simulink model "AirTableModel"  (R2021a)
settings: Solver=FixedStepAuto  StartTime=0.0  StopTime=endTime  FixedStep=dynamicsRate  RelTol=1e-3  EnableMultiTasking=on
InitFcn:
  | loadThrusterData
  | loadSensorData
values from neighbouring files (symbols this model uses):
  AccelIIR_Den = [1.000000000000000  -1.561018075800718   0.641351538057563]    [loadSensorData.m]
  AccelIIR_Num = [0.020083365564211   0.040166731128423   0.020083365564211]    [loadSensorData.m]
  cameraVec = [1 0 0]    [loadSensorData.m]
  controlRate = 0.025    [loadBusData.m]
  controlType = 1    [loadBusData.m]    (also in loadControlData.m = 2)
  dynamicsRate = 0.005    [loadBusData.m]
  finalRangeAttitude = [0 0 90]*dtr    [loadGuidanceData.m]
  finalRangeValue = 0.25    [loadGuidanceData.m]
  initialCovariance = diag([999999 999999 999999 999999 999999 999999])    [loadSensorData.m]
  initialNavState = [initialState + [0.01 -0.01 1e-3 0 0 1e-3]]    [loadSensorData.m]
  Kd = [x(4) x(5) 0 0 0 x(6)]    [executeSim.m]    (also in loadBusData.m = [500.0000  501.0938 0 0 0 18.4778]; loadControlData.m = [80 80 0 0 0 5] .*[.2 .2  0 0 0 .1]; planarPIDControl.m = [kd(1) 0 0; 0 kd(2) 0; 0 0 kd(3)])
  Ki = [x(7) x(8) 0 0 0 x(9)]    [executeSim.m]    (also in loadBusData.m = [1.0000    1.0313   0 0 0 58.1181]; loadControlData.m = [4  4  0 0 0 1] .*[1   1  0 0 0 .5]; planarPIDControl.m = [ki(1) 0 0; 0 ki(2) 0; 0 0 ki(3)])
  Kp = [x(1) x(2) 0 0 0 x(3)]    [executeSim.m]    (also in loadBusData.m = [500.0000  246.1321 0 0 0 50.1701]; loadControlData.m = [70 70 0 0 0 20].*[.2 .2  0 0 0 .25]; planarPIDControl.m = [kp(1) 0 0; 0 kp(2) 0; 0 0 kp(3)])
  M_Tracker_To_Body = [1 0 0; 0 1 0; 0 0 1]    [loadSensorData.m]
  measurementNoise = [1 .0873 0.0017 2].* [.01 1 1 .01]    [loadSensorData.m]
  processNoise = 0    [loadSensorData.m]
  R_Tracker_To_ECEF = [0 0 0]    [loadSensorData.m]
  rangeSensorAngBody = [0; 90*dtr; 180*dtr; 270*dtr]    [loadSensorData.m]
  rangeSensorFOV = [0*dtr; 0*dtr; 0*dtr; 0*dtr]    [loadSensorData.m]
  rangeSensorIdx = 1    [loadGuidanceData.m]
  SMGains = x    [executeSim.m]    (also in loadBusData.m = [2.0801    3.0489    8.9333    4.9881    3.0029    9.5293   ; loadControlData.m = [3.5078    3.9888    6.3119    1.8214    4.7749    7.3059   )
  useRangeGuid = 0    [loadGuidanceData.m]
  VelIIR_Den = [1.000000000000000  -1.944477657767094   0.945977936232282]    [loadSensorData.m]
  VelIIR_Num = [0.375069616296964   0.750139232593927   0.375069616296964]*1e-3    [loadSensorData.m]
  wallBounds = [wallA; wallB; wallC; wallD]    [loadSensorData.m]
undefined symbols (not defined in the file or in its folder): initialState, navType, PPGains, rangeSensorLocBody, refIdx, targetVec
libraries: simulink x25
(part 1 of 2)
settings Model: SimulationMode=external  Creator=Andy  LastModifiedBy=Andy
settings SolverCC: AlgebraicLoopSolver=TrustRegion  PositivePriorityOrder=on
settings DataIOCC: Decimation=5  SaveFormat=StructureWithTime  ReturnWorkspaceOutputs=off
settings OptimizationCC: EnhancedBackFolding=on  PassReuseOutputArgsAs=Individual arguments  ZeroExternalMemoryAtStartup=off  ZeroInternalMemoryAtStartup=off  MaxStackSize=1024  OptimizeBlockOrder=speed  DifferentSizesBufferReuse=on  OptimizationCustomize=off  EfficientTunableParamExpr=on
settings DebuggingCC: ParameterTunabilityLossMsg=error  SFMachineParentedDataDiag=warning  ArithmeticOperatorsInVariantConditions=warning
settings HardwareCC: ProdBitPerPointer=32  ProdBitPerSizeT=32  ProdBitPerPtrDiffT=32  ProdLargestAtomicInteger=Long  ProdLargestAtomicFloat=Double  ProdWordSize=32  ProdHWDeviceType=ARM Compatible->ARM Cortex
settings ModelReferenceCC: ModelReferenceNumInstancesAllowed=Single
settings SFSimCC: CustomCodeUndefinedFunction=UseInterfaceOnly  SimTargetLang=C++
settings RTWCC: SystemTargetFile=ert.tlc  HardwareBoard=Raspberry Pi  TLCOptions="-aInlineSetEventsForThisBaseRateFcn=TLC_TRUE -aSuppressMultiTaskScheduler=TLC_FALSE  -aRateBasedStepFcn=0"  GenCodeOnly=on  TemplateMakefile=ert_default_tmf  GenerateReport=on  Toolchain=GNU GCC Embedded Linux  BuildConfiguration=Faster Runs  IncludeHyperlinkInReport=on  LaunchReport=on  TargetLang=C++  GenerateTraceInfo=on  GenerateTraceReport=on  GenerateTraceReportSl=on  GenerateTraceReportSf=on  GenerateTraceReportEml=on
settings CodeAppCC: ForceParamTrailComments=on  IgnoreCustomStorageClasses=off  OperatorAnnotations=on  SimulinkDataObjDesc=on  SFDataObjDesc=on  InsertBlockDesc=on
settings ERTTargetCC: TargetLangStandard=C++03 (ISO)  UtilityFuncGeneration=Shared location  MatFileLogging=on  CodeInterfacePackaging=C++ class  SupportVariableSizeSignals=on  MultiInstanceErrorCode=Warning  RootIOFormat=Structure reference

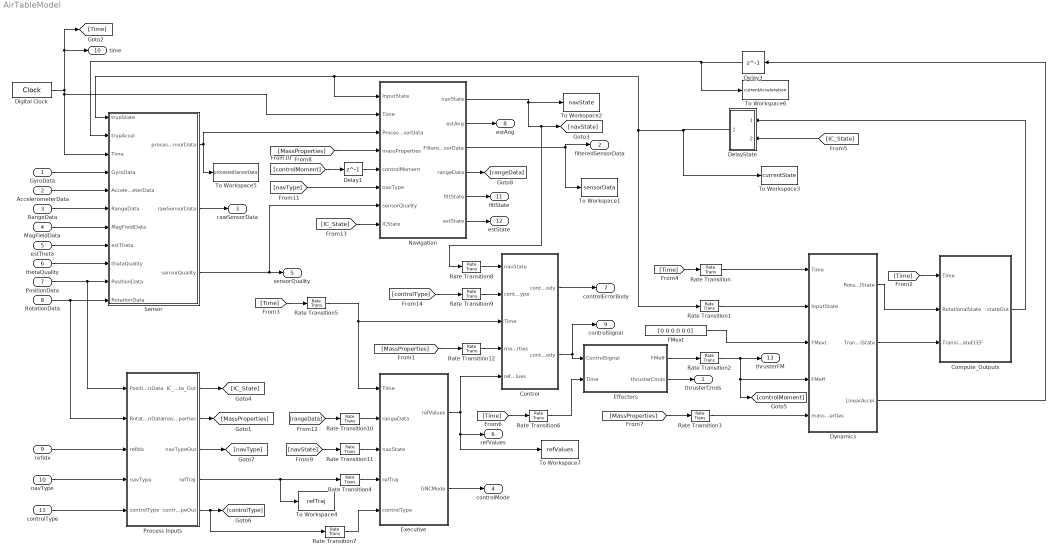
== system AirTableModel ==
  GyroData : Inport  Interpolate=off
  AccelerometerData : Inport  Port=2  Interpolate=off
  RangeData : Inport  Port=3  OutDataTypeStr=int32  Interpolate=off
  MagFieldData : Inport  Port=4  Interpolate=off
  estTheta : Inport  Port=5  OutDataTypeStr=double  PortDimensions=1  Interpolate=off
  thetaQuality : Inport  Port=6  OutDataTypeStr=double  PortDimensions=[1]  Interpolate=off
  PositionData : Inport  Port=7  OutDataTypeStr=double  PortDimensions=3  Interpolate=off
  RotationData : Inport  Port=8  OutDataTypeStr=double  PortDimensions=3  Interpolate=off
  refIdx : Inport  Port=9  OutDataTypeStr=uint8  PortDimensions=1  Interpolate=off
  navType : Inport  Port=10  OutDataTypeStr=uint8  PortDimensions=1  Interpolate=off
  controlType : Inport  Port=11  OutDataTypeStr=uint8  PortDimensions=1  Interpolate=off
  Compute_Outputs : Subsystem
  Control : Subsystem
  Delay1 : Delay  DelayLength=1
  Delay3 : Delay  DelayLength=1
  DelayState : Subsystem
  Digital Clock : DigitalClock  SampleTime=dynamicsRate
  Dynamics : Subsystem  TreatAsAtomicUnit=on  SystemSampleTime=dynamicsRate
      settings: MinAlgLoopOccurrences=on
  Effectors : Subsystem  TreatAsAtomicUnit=on
  Executive : Subsystem  TreatAsAtomicUnit=on  SystemSampleTime=controlRate
  FMext : Constant  Value=[0 0 0 0 0 0]
  Navigation : Subsystem
  Process Inputs : Subsystem
  Rate Transition{,1..3} (4 alike) : RateTransition  OutPortSampleTime=dynamicsRate
  Rate Transition{4..12} (9 alike) : RateTransition  OutPortSampleTime=controlRate
  Sensor : Subsystem
  To Workspace1 : ToWorkspace  VariableName=sensorData  SaveFormat=Timeseries  SampleTime=-1
  To Workspace2 : ToWorkspace  VariableName=navState  SaveFormat=Timeseries  SampleTime=-1
  To Workspace3 : ToWorkspace  VariableName=currentState  SaveFormat=Timeseries  SampleTime=-1
  To Workspace4 : ToWorkspace  VariableName=refTraj  SaveFormat=Timeseries  SampleTime=-1
  To Workspace5 : ToWorkspace  VariableName=processedSensorData  SaveFormat=Timeseries  SampleTime=-1
  To Workspace6 : ToWorkspace  VariableName=currentAcceleration  SaveFormat=Timeseries  SampleTime=-1
  To Workspace7 : ToWorkspace  VariableName=refValues  SaveFormat=Timeseries  SampleTime=-1
  thrusterCmds : Outport  VectorParamsAs1DForOutWhenUnconnected=off
  filteredSensorData : Outport  Port=2  OutDataTypeStr=double  VectorParamsAs1DForOutWhenUnconnected=off
  rawSensorData : Outport  Port=3  OutDataTypeStr=double  VectorParamsAs1DForOutWhenUnconnected=off
  controlMode : Outport  Port=4  VectorParamsAs1DForOutWhenUnconnected=off
  sensorQuality : Outport  Port=5  VectorParamsAs1DForOutWhenUnconnected=off
  refValues : Outport  Port=6  OutDataTypeStr=double  VectorParamsAs1DForOutWhenUnconnected=off
  controlErrorBody : Outport  Port=7  VectorParamsAs1DForOutWhenUnconnected=off
  estAng : Outport  Port=8  VectorParamsAs1DForOutWhenUnconnected=off
  controlSignal : Outport  Port=9  VectorParamsAs1DForOutWhenUnconnected=off
  time : Outport  Port=10  VectorParamsAs1DForOutWhenUnconnected=off
  filtState : Outport  Port=11  OutDataTypeStr=double  VectorParamsAs1DForOutWhenUnconnected=off
  estState : Outport  Port=12  OutDataTypeStr=double  VectorParamsAs1DForOutWhenUnconnected=off
  thrusterFM : Outport  Port=13  VectorParamsAs1DForOutWhenUnconnected=off
  wires:
  Digital Clock/1 -> Navigation/2(Time), Sensor/3(Time), [Time], time/1
  FMext/1 -> Dynamics/3(FMext)
  Control/2(controlSignalBody) -> controlSignal/1, Effectors/1(ControlSignal)
  Dynamics/1(RotationalState) -> Compute_Outputs/2(RotationalState)
  Rate Transition/1 -> Dynamics/1(Time)
  Rate Transition1/1 -> Dynamics/2(InputState)
  Effectors/1(FMeff) -> Rate Transition2/1
  Rate Transition2/1 -> [controlMoment], Dynamics/4(FMeff), thrusterFM/1
  Rate Transition3/1 -> Dynamics/5(massProperties)
  Rate Transition5/1 -> Executive/1(Time), Control/3(Time)
  Rate Transition6/1 -> Effectors/2(Time)
  Dynamics/2(TranslationalState) -> Compute_Outputs/3(TranslationalStateECEF)
  Compute_Outputs/1(stateOut) -> DelayState/1(In4)
  [IC_State] -> DelayState/2(In12)
  DelayState/1(Out4) -> To Workspace3/1, Rate Transition1/1, Navigation/1(InputState), Sensor/1(trueState)
  [Time] -> Compute_Outputs/1(Time)
  Rate Transition8/1 -> Control/1(navState)
  Effectors/2(thrusterCmds) -> thrusterCmds/1
  GyroData/1 -> Sensor/4(GyroData)
  AccelerometerData/1 -> Sensor/5(AccelerometerData)
  RangeData/1 -> Sensor/6(RangeData)
  Executive/1(refValues) -> Control/5(refValues), To Workspace7/1, refValues/1
  Rate Transition11/1 -> Executive/3(navState)
  [Time] -> Rate Transition5/1
  MagFieldData/1 -> Sensor/7(MagFieldData)
  Navigation/1(navState) -> Rate Transition8/1, [navState], To Workspace2/1
  [Time] -> Rate Transition/1
  [Time] -> Rate Transition6/1
  Rate Transition12/1 -> Control/4(massProperties)
  [MassProperties] -> Rate Transition12/1
  [MassProperties] -> Rate Transition3/1
  estTheta/1 -> Sensor/8(estTheta)
  thetaQuality/1 -> Sensor/9(thetaQuality)
  PositionData/1 -> Sensor/10(PositionData), Process Inputs/1(PositionData)
  RotationData/1 -> Process Inputs/2(RotationData), Sensor/11(RotationData)
  Sensor/1(processedSensorData) -> Navigation/3(ProcessedSensorData), To Workspace5/1
  Sensor/2(rawSensorData) -> rawSensorData/1
  [navState] -> Rate Transition11/1
  Rate Transition4/1 -> Executive/4(refTraj)
  Sensor/3(sensorQuality) -> sensorQuality/1, Navigation/7(sensorQuality)
  Control/1(controlErrorBody) -> controlErrorBody/1
  Navigation/2(estAng) -> estAng/1
  Dynamics/3(LinearAccel) -> Delay3/1
  Delay3/1 -> To Workspace6/1, Sensor/2(trueAccel)
  Navigation/3(FilteredSensorData) -> To Workspace1/1, filteredSensorData/1
  [MassProperties] -> Navigation/4(massProperties)
  [controlMoment] -> Delay1/1
  Delay1/1 -> Navigation/5(controlMoment)
  Navigation/5(flttState) -> filtState/1
  Navigation/6(estState) -> estState/1
  [navType] -> Navigation/6(navType)
  Process Inputs/4(refTraj) -> To Workspace4/1, Rate Transition4/1
  refIdx/1 -> Process Inputs/3(refIdx)
  navType/1 -> Process Inputs/4(navType)
  Process Inputs/2(massProperties) -> [MassProperties]
  Process Inputs/3(navTypeOut) -> [navType]
  Process Inputs/1(IC_State_Out) -> [IC_State]
  Rate Transition10/1 -> Executive/2(rangeData)
  Navigation/4(rangeData) -> [rangeData]
  [rangeData] -> Rate Transition10/1
  Executive/2(GNCMode) -> controlMode/1
  [IC_State] -> Navigation/8(ICState)
  [controlType] -> Rate Transition9/1
  controlType/1 -> Process Inputs/5(controlType)
  Process Inputs/5(controlTypeOut) -> Rate Transition7/1, [controlType]
  Rate Transition7/1 -> Executive/5(controlType)
  Rate Transition9/1 -> Control/2(controlType)

== system AirTableModel/Compute_Outputs ==
  Time : Inport
  RotationalState : Inport  Port=2
  TranslationalStateECEF : Inport  Port=3
  Bus Creator2 : BusCreator  Inputs=2  OutDataTypeStr=Bus: TranStateBodyBus
      settings: InheritFromInputs=off
  Bus Creator3 : BusCreator  Inputs=3  OutDataTypeStr=Bus: FullStateBus
      settings: InheritFromInputs=off
  Bus Selector : BusSelector  OutputSignals=ECEF_To_Body_Quat
  Bus Selector1 : BusSelector  OutputSignals=R_Sys_ECEF,V_Sys_ECEF
  Rotate_Vector : MATLAB Function  TreatAsAtomicUnit=on
  Rotate_Vector1 : MATLAB Function  TreatAsAtomicUnit=on
  Terminator1 : Terminator
  Terminator2 : Terminator
  To Workspace1 : ToWorkspace  VariableName=stateOutBus  SaveFormat=Timeseries  SampleTime=-1
  computeRangeData : Subsystem  Commented=on
  stateOut : Outport  VectorParamsAs1DForOutWhenUnconnected=off
  wires:
  RotationalState/1 -> Bus Creator3/1, Bus Selector/1
  Rotate_Vector/1(vOut) -> Bus Creator2/1
  Rotate_Vector1/1(vOut) -> Bus Creator2/2
  TranslationalStateECEF/1 -> Bus Creator3/2, Bus Selector1/1
  Bus Selector1/1 -> Rotate_Vector/1(vIn)  "<R_Sys_ECEF>"
  Bus Creator3/1 -> stateOut/1, To Workspace1/1, computeRangeData/2(In1)
  Time/1 -> computeRangeData/1(Time)
  Bus Selector/1 -> Rotate_Vector1/2(quat), [ECEF_To_Body_Quat]  "<ECEF_To_Body_Quat>"
  [ECEF_To_Body_Quat] -> Rotate_Vector/2(quat)
  Bus Selector1/2 -> Rotate_Vector1/1(vIn)  "<V_Sys_ECEF>"
  computeRangeData/1(range) -> Terminator1/1
  computeRangeData/2(rangeArray) -> Terminator2/1
  Bus Creator2/1 -> Bus Creator3/3

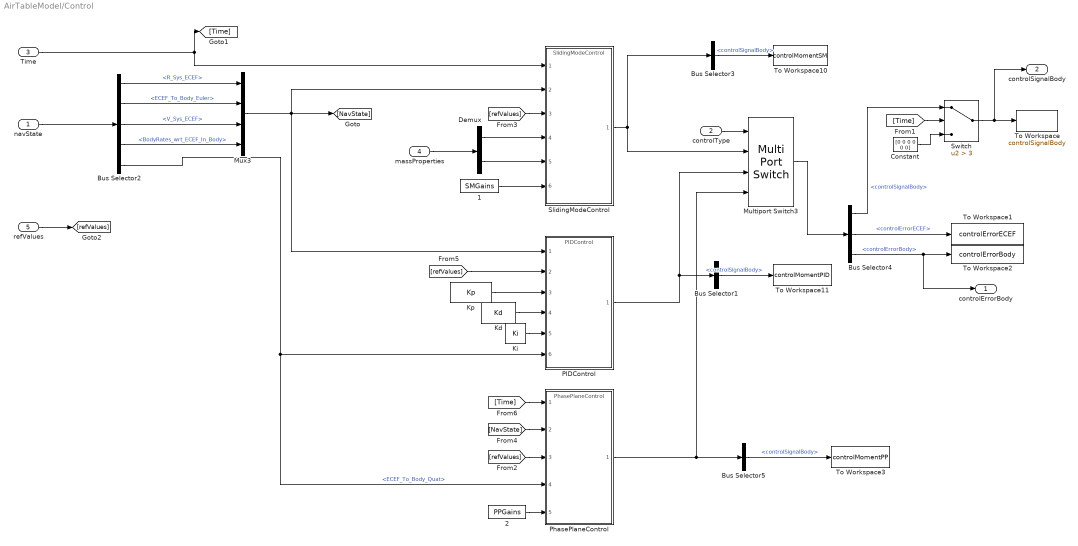
== system AirTableModel/Control ==
  navState : Inport
  controlType : Inport  Port=2
  Time : Inport  Port=3
  massProperties : Inport  Port=4
  refValues : Inport  Port=5
  " 1" : Constant  Value=SMGains
  " 2" : Constant  Value=PPGains
  Bus Selector1 : BusSelector  OutputSignals=controlSignalBody
  Bus Selector2 : BusSelector  OutputSignals=TranState_ECEF.R_Sys_ECEF,RotState_Body_ECEF.ECEF_To_Body_Euler,TranState_ECEF.V_Sys_ECEF,RotState_Body_ECEF.BodyRates_wrt_ECEF_In_Body,RotState_Body_ECEF.ECEF_To_Body_Quat
  Bus Selector3 : BusSelector  OutputSignals=controlSignalBody
  Bus Selector4 : BusSelector  OutputSignals=controlSignalBody,controlErrorECEF,controlErrorBody
  Bus Selector5 : BusSelector  OutputSignals=controlSignalBody
  Constant : Constant  Value=[0 0 0 0 0 0]
  Demux : Demux  Outputs=2
  Kd : Constant  Value=Kd
  Ki : Constant  Value=Ki
  Kp : Constant  Value=Kp
  Multiport Switch3 : MultiPortSwitch
  Mux3 : Mux
  PIDControl : ModelReference  ModelNameDialog=PIDControl  SimulationMode=Normal  ModelReferenceVersion=6.1
  PhasePlaneControl : ModelReference  ModelNameDialog=PhasePlaneControl  SimulationMode=Normal  ModelReferenceVersion=6.20
  SlidingModeControl : ModelReference  ModelNameDialog=SlidingModeControl  SimulationMode=Normal  ModelReferenceVersion=6.1
  Switch : Switch  Criteria=u2 > Threshold  Threshold=3
  To Workspace : ToWorkspace  VariableName=controlSignalBody  SaveFormat=Timeseries  SampleTime=-1
  To Workspace1 : ToWorkspace  VariableName=controlErrorECEF  SaveFormat=Timeseries  SampleTime=-1
  To Workspace10 : ToWorkspace  VariableName=controlMomentSM  SaveFormat=Timeseries  SampleTime=-1
  To Workspace11 : ToWorkspace  VariableName=controlMomentPID  SaveFormat=Timeseries  SampleTime=-1
  To Workspace2 : ToWorkspace  VariableName=controlErrorBody  SaveFormat=Timeseries  SampleTime=-1
  To Workspace3 : ToWorkspace  VariableName=controlMomentPP  SaveFormat=Timeseries  SampleTime=-1
  controlErrorBody : Outport  VectorParamsAs1DForOutWhenUnconnected=off
  controlSignalBody : Outport  Port=2  VectorParamsAs1DForOutWhenUnconnected=off
  wires:
  Mux3/1 -> PIDControl/1, [NavState], SlidingModeControl/2
  navState/1 -> Bus Selector2/1
  Bus Selector2/1 -> Mux3/1  "<R_Sys_ECEF>"
  Bus Selector2/2 -> Mux3/2  "<ECEF_To_Body_Euler>"
  Bus Selector2/3 -> Mux3/3  "<V_Sys_ECEF>"
  Bus Selector2/4 -> Mux3/4  "<BodyRates_wrt_ECEF_In_Body>"
  Kp/1 -> PIDControl/3
  Kd/1 -> PIDControl/4
  Ki/1 -> PIDControl/5
  Demux/2 -> SlidingModeControl/5
  SlidingModeControl/1 -> Bus Selector3/1, Multiport Switch3/2
  controlType/1 -> Multiport Switch3/1
  PIDControl/1 -> Bus Selector1/1, Multiport Switch3/3
  Multiport Switch3/1 -> Bus Selector4/1
  Bus Selector4/1 -> Switch/1  "<controlSignalBody>"
  Bus Selector4/2 -> To Workspace1/1  "<controlErrorECEF>"
  Bus Selector4/3 -> controlErrorBody/1, To Workspace2/1  "<controlErrorBody>"
  Bus Selector1/1 -> To Workspace11/1  "<controlSignalBody>"
  Bus Selector3/1 -> To Workspace10/1  "<controlSignalBody>"
  " 1"/1 -> SlidingModeControl/6
  Demux/1 -> SlidingModeControl/4
  massProperties/1 -> Demux/1
  Time/1 -> [Time], SlidingModeControl/1
  [refValues] -> SlidingModeControl/3
  [refValues] -> PIDControl/2
  Bus Selector2/5 -> PIDControl/6, PhasePlaneControl/4  "<ECEF_To_Body_Quat>"
  [Time] -> Switch/2
  Switch/1 -> controlSignalBody/1, To Workspace/1
  Constant/1 -> Switch/3
  refValues/1 -> [refValues]
  [refValues] -> PhasePlaneControl/3
  [NavState] -> PhasePlaneControl/2
  " 2"/1 -> PhasePlaneControl/5
  [Time] -> PhasePlaneControl/1
  Bus Selector5/1 -> To Workspace3/1  "<controlSignalBody>"
  PhasePlaneControl/1 -> Multiport Switch3/4, Bus Selector5/1

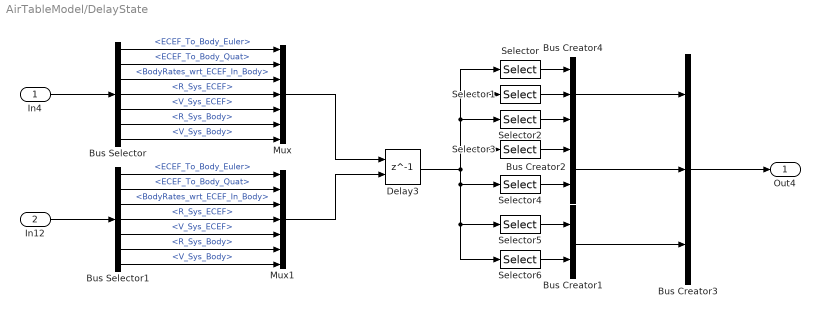
== system AirTableModel/DelayState ==
  In4 : Inport
  In12 : Inport  Port=2
  Bus Creator1 : BusCreator  Inputs=2  OutDataTypeStr=Bus: TranStateBodyBus
      settings: InheritFromInputs=off
  Bus Creator2 : BusCreator  Inputs=2  OutDataTypeStr=Bus: TranStateECEFBus
      settings: InheritFromInputs=off
  Bus Creator3 : BusCreator  Inputs=3  OutDataTypeStr=Bus: FullStateBus
      settings: InheritFromInputs=off
  Bus Creator4 : BusCreator  Inputs=3  OutDataTypeStr=Bus: RotStateBodyECEFBus
      settings: InheritFromInputs=off
  Bus Selector : BusSelector  OutputSignals=RotState_Body_ECEF.ECEF_To_Body_Euler,RotState_Body_ECEF.ECEF_To_Body_Quat,RotState_Body_ECEF.BodyRates_wrt_ECEF_In_Body,TranState_ECEF.R_Sys_ECEF,TranState_ECEF.V_Sys_ECEF,TranState_Body.R_Sys_Body,TranState_Body.V_Sys_Body
  Bus Selector1 : BusSelector  OutputSignals=RotState_Body_ECEF.ECEF_To_Body_Euler,RotState_Body_ECEF.ECEF_To_Body_Quat,RotState_Body_ECEF.BodyRates_wrt_ECEF_In_Body,TranState_ECEF.R_Sys_ECEF,TranState_ECEF.V_Sys_ECEF,TranState_Body.R_Sys_Body,TranState_Body.V_Sys_Body
  Delay3 : Delay  DelayLength=1  InitialConditionSource=Input port
      settings: InputPortMap=u0,p4
  Mux : Mux  Inputs=7
  Mux1 : Mux  Inputs=7
  Selector : Selector  InputPortWidth=22  IndexOptions=Index vector (dialog)  Indices=[1:3]  OutputSizes=1
  Selector1 : Selector  InputPortWidth=22  IndexOptions=Index vector (dialog)  Indices=[4:7]  OutputSizes=1
  Selector2 : Selector  InputPortWidth=22  IndexOptions=Index vector (dialog)  Indices=[8:10]  OutputSizes=1
  Selector3 : Selector  InputPortWidth=22  IndexOptions=Index vector (dialog)  Indices=[11:13]  OutputSizes=1
  Selector4 : Selector  InputPortWidth=22  IndexOptions=Index vector (dialog)  Indices=[14:16]  OutputSizes=1
  Selector5 : Selector  InputPortWidth=22  IndexOptions=Index vector (dialog)  Indices=[17:19]  OutputSizes=1
  Selector6 : Selector  InputPortWidth=22  IndexOptions=Index vector (dialog)  Indices=[20:22]  OutputSizes=1
  Out4 : Outport  VectorParamsAs1DForOutWhenUnconnected=off
  wires:
  Bus Creator3/1 -> Out4/1
  Bus Creator1/1 -> Bus Creator3/3
  Bus Creator2/1 -> Bus Creator3/2
  Bus Creator4/1 -> Bus Creator3/1
  In4/1 -> Bus Selector/1
  Bus Selector/1 -> Mux/1  "<ECEF_To_Body_Euler>"
  Bus Selector/2 -> Mux/2  "<ECEF_To_Body_Quat>"
  Bus Selector/3 -> Mux/3  "<BodyRates_wrt_ECEF_In_Body>"
  Bus Selector/4 -> Mux/4  "<R_Sys_ECEF>"
  Bus Selector/5 -> Mux/5  "<V_Sys_ECEF>"
  Bus Selector/6 -> Mux/6  "<R_Sys_Body>"
  Bus Selector/7 -> Mux/7  "<V_Sys_Body>"
  Bus Selector1/4 -> Mux1/4  "<R_Sys_ECEF>"
  Bus Selector1/2 -> Mux1/2  "<ECEF_To_Body_Quat>"
  Bus Selector1/1 -> Mux1/1  "<ECEF_To_Body_Euler>"
  In12/1 -> Bus Selector1/1
  Bus Selector1/6 -> Mux1/6  "<R_Sys_Body>"
  Bus Selector1/5 -> Mux1/5  "<V_Sys_ECEF>"
  Bus Selector1/7 -> Mux1/7  "<V_Sys_Body>"
  Bus Selector1/3 -> Mux1/3  "<BodyRates_wrt_ECEF_In_Body>"
  Mux/1 -> Delay3/1
  Mux1/1 -> Delay3/2
  Selector/1 -> Bus Creator4/1
  Selector1/1 -> Bus Creator4/2
  Selector2/1 -> Bus Creator4/3
  Selector3/1 -> Bus Creator2/1
  Selector4/1 -> Bus Creator2/2
  Selector5/1 -> Bus Creator1/1
  Selector6/1 -> Bus Creator1/2
  Delay3/1 -> Selector/1, Selector1/1, Selector2/1, Selector3/1, Selector4/1, Selector5/1, Selector6/1

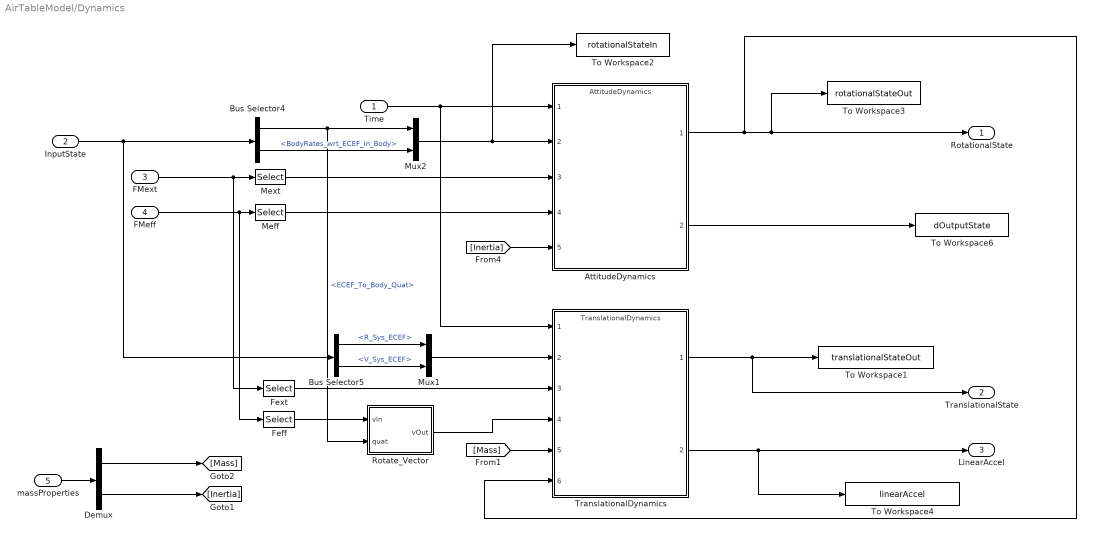
== system AirTableModel/Dynamics ==
  Time : Inport
  InputState : Inport  Port=2
  FMext : Inport  Port=3
  FMeff : Inport  Port=4
  massProperties : Inport  Port=5
  AttitudeDynamics : ModelReference  ModelNameDialog=AttitudeDynamics  SimulationMode=Normal  ModelReferenceVersion=1.386
  Bus Selector4 : BusSelector  OutputSignals=RotState_Body_ECEF.ECEF_To_Body_Quat,RotState_Body_ECEF.BodyRates_wrt_ECEF_In_Body
  Bus Selector5 : BusSelector  OutputSignals=TranState_ECEF.R_Sys_ECEF,TranState_ECEF.V_Sys_ECEF
  Demux : Demux  Outputs=2
  Feff : Selector  InputPortWidth=6  IndexOptions=Index vector (dialog)  Indices=[1:3]  OutputSizes=1
  Fext : Selector  InputPortWidth=6  IndexOptions=Index vector (dialog)  Indices=[1:3]  OutputSizes=1
  Meff : Selector  InputPortWidth=6  IndexOptions=Index vector (dialog)  Indices=[4:6]  OutputSizes=1
  Mext : Selector  InputPortWidth=6  IndexOptions=Index vector (dialog)  Indices=[4:6]  OutputSizes=1
  Mux1 : Mux  Inputs=2
  Mux2 : Mux  Inputs=2
  Rotate_Vector : MATLAB Function  TreatAsAtomicUnit=on
  To Workspace1 : ToWorkspace  VariableName=translationalStateOut  SaveFormat=Timeseries  SampleTime=-1
  To Workspace2 : ToWorkspace  VariableName=rotationalStateIn  SaveFormat=Timeseries  SampleTime=-1
  To Workspace3 : ToWorkspace  VariableName=rotationalStateOut  SaveFormat=Timeseries  SampleTime=-1
  To Workspace4 : ToWorkspace  VariableName=linearAccel  SaveFormat=Timeseries  SampleTime=-1
  To Workspace6 : ToWorkspace  VariableName=dOutputState  SaveFormat=Timeseries  SampleTime=-1
  TranslationalDynamics : ModelReference  ModelNameDialog=TranslationalDynamics  SimulationMode=Normal  ModelReferenceVersion=1.366
  RotationalState : Outport  VectorParamsAs1DForOutWhenUnconnected=off
  TranslationalState : Outport  Port=2  VectorParamsAs1DForOutWhenUnconnected=off
  LinearAccel : Outport  Port=3  VectorParamsAs1DForOutWhenUnconnected=off
  wires:
  Time/1 -> AttitudeDynamics/1, TranslationalDynamics/1
  FMext/1 -> Mext/1, Fext/1
  Mext/1 -> AttitudeDynamics/3
  Fext/1 -> TranslationalDynamics/3
  FMeff/1 -> Feff/1, Meff/1
  Meff/1 -> AttitudeDynamics/4
  AttitudeDynamics/2 -> To Workspace6/1
  AttitudeDynamics/1 -> RotationalState/1, To Workspace3/1, TranslationalDynamics/6
  TranslationalDynamics/1 -> TranslationalState/1, To Workspace1/1
  InputState/1 -> Bus Selector5/1, Bus Selector4/1
  Bus Selector4/1 -> Rotate_Vector/2(quat), Mux2/1  "<ECEF_To_Body_Quat>"
  Bus Selector4/2 -> Mux2/2  "<BodyRates_wrt_ECEF_In_Body>"
  Mux1/1 -> TranslationalDynamics/2
  Mux2/1 -> To Workspace2/1, AttitudeDynamics/2
  Bus Selector5/1 -> Mux1/1  "<R_Sys_ECEF>"
  Bus Selector5/2 -> Mux1/2  "<V_Sys_ECEF>"
  massProperties/1 -> Demux/1
  [Inertia] -> AttitudeDynamics/5
  [Mass] -> TranslationalDynamics/5
  Demux/1 -> [Mass]
  Demux/2 -> [Inertia]
  TranslationalDynamics/2 -> To Workspace4/1, LinearAccel/1
  Feff/1 -> Rotate_Vector/1(vIn)
  Rotate_Vector/1(vOut) -> TranslationalDynamics/4

== system AirTableModel/Effectors ==
  ControlSignal : Inport
  Time : Inport  Port=2
  Mux4 : Mux  Inputs=2
  ReactionWheel : ModelReference  ModelNameDialog=ReactionWheel0  SimulationMode=Normal  ModelReferenceVersion=1.304
  Selector1 : Selector  InputPortWidth=6  IndexOptions=Index vector (dialog)  Indices=[6]  OutputSizes=1
  ThrusterModel : ModelReference  ModelNameDialog=ThrusterModel0  SimulationMode=Normal  ModelReferenceVersion=1.341
  To Workspace1 : ToWorkspace  VariableName=wheelMoment  SaveFormat=Timeseries  SampleTime=-1
  To Workspace2 : ToWorkspace  VariableName=wheelOut  SaveFormat=Timeseries  SampleTime=-1
  To Workspace3 : ToWorkspace  VariableName=thrusterOnTimes  SaveFormat=Timeseries  SampleTime=-1
  To Workspace4 : ToWorkspace  VariableName=thrusterOnPulse  SaveFormat=Timeseries  SampleTime=-1
  To Workspace5 : ToWorkspace  VariableName=thrusterOut  SaveFormat=Timeseries  SampleTime=-1
  To Workspace6 : ToWorkspace  VariableName=thrusterCmds  SaveFormat=Timeseries  SampleTime=-1
  FMeff : Outport  VectorParamsAs1DForOutWhenUnconnected=off
  thrusterCmds : Outport  Port=2  VectorParamsAs1DForOutWhenUnconnected=off
  wires:
  Selector1/1 -> ReactionWheel/2
  ControlSignal/1 -> ThrusterModel/1, Selector1/1
  Time/1 -> ThrusterModel/2, ReactionWheel/1
  Mux4/1 -> FMeff/1, To Workspace5/1
  ThrusterModel/3 -> To Workspace6/1, thrusterCmds/1
  ReactionWheel/1 -> To Workspace1/1
  ReactionWheel/2 -> To Workspace2/1
  ThrusterModel/2 -> Mux4/2
  ThrusterModel/1 -> Mux4/1
  ThrusterModel/4 -> To Workspace3/1
  ThrusterModel/5 -> To Workspace4/1

== system AirTableModel/Executive ==
  Time : Inport
  rangeData : Inport  Port=2
  navState : Inport  Port=3
  refTraj : Inport  Port=4
  controlType : Inport  Port=5
  Constant : Constant
  Delay : Delay  DelayLength=1  InitialConditionSource=Input port  InitialCondition=0
      settings: InputPortMap=u0,p4
  Guidance : Subsystem
  MATLAB Function : MATLAB Function  TreatAsAtomicUnit=on
  To Workspace2 : ToWorkspace  VariableName=GNCMode  SaveFormat=Timeseries  SampleTime=-1
  UseRangeGuid : Constant  Value=useRangeGuid
  refValues : Outport  VectorParamsAs1DForOutWhenUnconnected=off
  GNCMode : Outport  Port=2  VectorParamsAs1DForOutWhenUnconnected=off
  wires:
  Delay/1 -> MATLAB Function/4(inGNCMode)
  MATLAB Function/1(outGNCMode) -> To Workspace2/1, GNCMode/1, Guidance/3(GNCMode), Delay/1
  Constant/1 -> Delay/2
  refTraj/1 -> Guidance/2(refTraj), MATLAB Function/2(refTraj)
  navState/1 -> Guidance/1(navState), MATLAB Function/1(navState)
  Time/1 -> Guidance/4(Time)
  controlType/1 -> Guidance/5(controlType)
  rangeData/1 -> Guidance/6(rangeData)  "rangeData"
  Guidance/1(Out1) -> refValues/1
  UseRangeGuid/1 -> MATLAB Function/3(useRangeGuid)

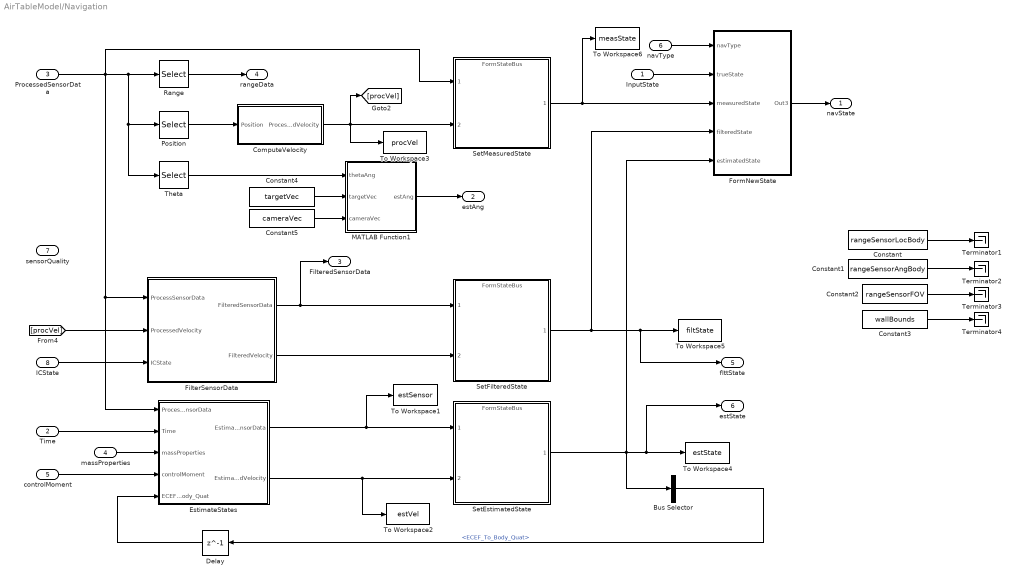
== system AirTableModel/Navigation ==
  InputState : Inport
  Time : Inport  Port=2
  ProcessedSensorData : Inport  Port=3
  massProperties : Inport  Port=4
  controlMoment : Inport  Port=5
  navType : Inport  Port=6
  sensorQuality : Inport  Port=7
  ICState : Inport  Port=8
  Bus Selector : BusSelector  OutputSignals=RotState_Body_ECEF.ECEF_To_Body_Quat
  ComputeVelocity : Subsystem
  Constant : Constant  Value=rangeSensorLocBody
  Constant1 : Constant  Value=rangeSensorAngBody
  Constant2 : Constant  Value=rangeSensorFOV
  Constant3 : Constant  Value=wallBounds
  Constant4 : Constant  Value=targetVec
  Constant5 : Constant  Value=cameraVec
  Delay : Delay  DelayLength=1  InitialCondition=[1 0 0 0]
  EstimateStates : Subsystem
  FilterSensorData : Subsystem
  FormNewState : Subsystem
  MATLAB Function1 : MATLAB Function  TreatAsAtomicUnit=on
  Position : Selector  InputPortWidth=20  IndexOptions=Index vector (dialog)  Indices=[15:17]  OutputSizes=1
  Range : Selector  InputPortWidth=20  IndexOptions=Index vector (dialog)  Indices=[7:10]  OutputSizes=1
  SetEstimatedState : ModelReference  ModelNameDialog=FormStateBus  SimulationMode=Normal  ModelReferenceVersion=1.29
  SetFilteredState : ModelReference  ModelNameDialog=FormStateBus  SimulationMode=Normal  ModelReferenceVersion=1.29
  SetMeasuredState : ModelReference  ModelNameDialog=FormStateBus  SimulationMode=Normal  ModelReferenceVersion=1.29
  Terminator{1..4} (4 alike) : Terminator
  Theta : Selector  InputPortWidth=20  IndexOptions=Index vector (dialog)  Indices=[14]  OutputSizes=1
  To Workspace1 : ToWorkspace  VariableName=estSensor  SaveFormat=Timeseries  SampleTime=-1
  To Workspace2 : ToWorkspace  VariableName=estVel  SaveFormat=Timeseries  SampleTime=-1
  To Workspace3 : ToWorkspace  VariableName=procVel  SaveFormat=Timeseries  SampleTime=-1
  To Workspace4 : ToWorkspace  VariableName=estState  SaveFormat=Timeseries  SampleTime=-1
  To Workspace5 : ToWorkspace  VariableName=filtState  SaveFormat=Timeseries  SampleTime=-1
  To Workspace6 : ToWorkspace  VariableName=measState  SaveFormat=Timeseries  SampleTime=-1
  navState : Outport  VectorParamsAs1DForOutWhenUnconnected=off
  estAng : Outport  Port=2  VectorParamsAs1DForOutWhenUnconnected=off
  FilteredSensorData : Outport  Port=3  VectorParamsAs1DForOutWhenUnconnected=off
  rangeData : Outport  Port=4  VectorParamsAs1DForOutWhenUnconnected=off
  flttState : Outport  Port=5  VectorParamsAs1DForOutWhenUnconnected=off
  estState : Outport  Port=6  VectorParamsAs1DForOutWhenUnconnected=off
  wires:
  InputState/1 -> FormNewState/2(trueState)
  FormNewState/1(Out3) -> navState/1
  Range/1 -> rangeData/1
  Constant3/1 -> Terminator4/1
  Constant2/1 -> Terminator3/1
  Constant1/1 -> Terminator2/1
  Constant/1 -> Terminator1/1
  Theta/1 -> MATLAB Function1/1(thetaAng)
  Constant4/1 -> MATLAB Function1/2(targetVec)
  MATLAB Function1/1(estAng) -> estAng/1
  Constant5/1 -> MATLAB Function1/3(cameraVec)
  ComputeVelocity/1(ProcessedVelocity) -> To Workspace3/1, SetMeasuredState/2, [procVel]
  Position/1 -> ComputeVelocity/1(Position)
  ProcessedSensorData/1 -> EstimateStates/1(ProcessSensorData), FilterSensorData/1(ProcessSensorData), SetMeasuredState/1, Theta/1, Position/1, Range/1
  [procVel] -> FilterSensorData/2(ProcessedVelocity)
  FilterSensorData/1(FilteredSensorData) -> FilteredSensorData/1, SetFilteredState/1
  FilterSensorData/2(FilteredVelocity) -> SetFilteredState/2
  SetMeasuredState/1 -> To Workspace6/1, FormNewState/3(measuredState)
  SetFilteredState/1 -> flttState/1, To Workspace5/1, FormNewState/4(filteredState)
  massProperties/1 -> EstimateStates/3(massProperties)
  controlMoment/1 -> EstimateStates/4(controlMoment)
  SetEstimatedState/1 -> Bus Selector/1, FormNewState/5(estimatedState), estState/1, To Workspace4/1
  Bus Selector/1 -> Delay/1  "<ECEF_To_Body_Quat>"
  Delay/1 -> EstimateStates/5(ECEF_To_Body_Quat)
  Time/1 -> EstimateStates/2(Time)
  EstimateStates/1(EstimatedSensorData) -> To Workspace1/1, SetEstimatedState/1
  EstimateStates/2(EstimatedVelocity) -> To Workspace2/1, SetEstimatedState/2
  navType/1 -> FormNewState/1(navType)
  ICState/1 -> FilterSensorData/3(ICState)

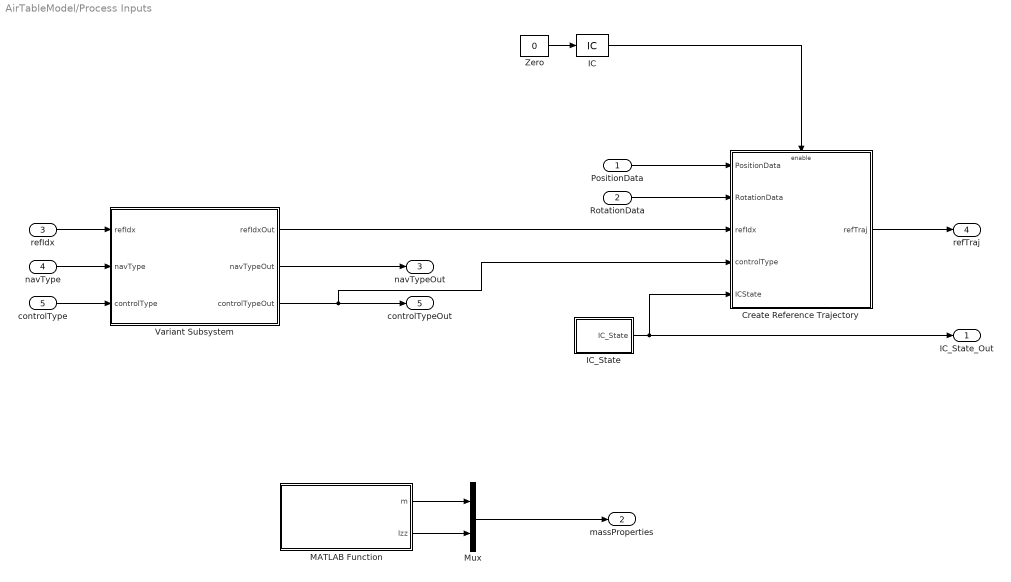
== system AirTableModel/Process Inputs ==
  PositionData : Inport
  RotationData : Inport  Port=2
  refIdx : Inport  Port=3  OutDataTypeStr=uint8  PortDimensions=1
  navType : Inport  Port=4  OutDataTypeStr=uint8  PortDimensions=1
  controlType : Inport  Port=5  OutDataTypeStr=uint8  PortDimensions=1
  Create Reference Trajectory : Subsystem  TreatAsAtomicUnit=on
  IC : InitialCondition
  IC_State : Subsystem
  MATLAB Function : MATLAB Function  TreatAsAtomicUnit=on
  Mux : Mux  Inputs=2
  Variant Subsystem : Subsystem  Variant=on
  Zero : Constant  Value=0
  IC_State_Out : Outport
  massProperties : Outport  Port=2
  navTypeOut : Outport  Port=3
  refTraj : Outport  Port=4
  controlTypeOut : Outport  Port=5
  wires:
  MATLAB Function/2(Izz) -> Mux/2
  IC/1 -> Create Reference Trajectory/Enable
  IC_State/1(IC_State) -> Create Reference Trajectory/5(ICState), IC_State_Out/1
  MATLAB Function/1(m) -> Mux/1
  PositionData/1 -> Create Reference Trajectory/1(PositionData)
  Variant Subsystem/2(navTypeOut) -> navTypeOut/1
  refIdx/1 -> Variant Subsystem/1(refIdx)
  Zero/1 -> IC/1
  navType/1 -> Variant Subsystem/2(navType)
  Variant Subsystem/1(refIdxOut) -> Create Reference Trajectory/3(refIdx)
  RotationData/1 -> Create Reference Trajectory/2(RotationData)
  Create Reference Trajectory/1(refTraj) -> refTraj/1
  Mux/1 -> massProperties/1
  controlType/1 -> Variant Subsystem/3(controlType)
  Variant Subsystem/3(controlTypeOut) -> Create Reference Trajectory/4(controlType), controlTypeOut/1

== system AirTableModel/Sensor ==
  note: This is a Variant Subsystem.
      | The version is chosen through the VSS_MODE workspace variable
  trueState : Inport  OutDataTypeStr=double
  trueAccel : Inport  Port=2  OutDataTypeStr=double
  Time : Inport  Port=3  OutDataTypeStr=double
  GyroData : Inport  Port=4  OutDataTypeStr=double
  AccelerometerData : Inport  Port=5  OutDataTypeStr=double
  RangeData : Inport  Port=6  OutDataTypeStr=int32
  MagFieldData : Inport  Port=7  OutDataTypeStr=double
  estTheta : Inport  Port=8
  thetaQuality : Inport  Port=9
  PositionData : Inport  Port=10
  RotationData : Inport  Port=11
  Variant Subsystem : Subsystem  Variant=on
  processedSensorData : Outport  OutDataTypeStr=double  VectorParamsAs1DForOutWhenUnconnected=off
  rawSensorData : Outport  Port=2  OutDataTypeStr=double  VectorParamsAs1DForOutWhenUnconnected=off
  sensorQuality : Outport  Port=3  VectorParamsAs1DForOutWhenUnconnected=off
  wires:
  trueState/1 -> Variant Subsystem/1(trueState)
  GyroData/1 -> Variant Subsystem/4(GyroData)
  AccelerometerData/1 -> Variant Subsystem/5(AccelerometerData)
  RangeData/1 -> Variant Subsystem/6(RangeData)
  Variant Subsystem/1(ProcessedSensorData) -> processedSensorData/1
  MagFieldData/1 -> Variant Subsystem/7(MagFieldData)
  Variant Subsystem/2(RawSensorData) -> rawSensorData/1
  Variant Subsystem/3(sensorQuality) -> sensorQuality/1
  estTheta/1 -> Variant Subsystem/8(estTheta)
  thetaQuality/1 -> Variant Subsystem/9(thetaQuality)
  PositionData/1 -> Variant Subsystem/10(PositionData)
  RotationData/1 -> Variant Subsystem/11(RotationData)
  Time/1 -> Variant Subsystem/3(Time)
  trueAccel/1 -> Variant Subsystem/2(trueAccel)

== system AirTableModel/Compute_Outputs/computeRangeData ==
  Time : Inport
  In1 : Inport  Port=2
  Constant : Constant  Value=rangeSensorLocBody
  Constant1 : Constant  Value=rangeSensorAngBody
  Constant2 : Constant  Value=rangeSensorFOV
  Constant3 : Constant  Value=wallBounds
  MATLAB Function1 : MATLAB Function  TreatAsAtomicUnit=on
  range : Outport  VectorParamsAs1DForOutWhenUnconnected=off
  rangeArray : Outport  Port=2  VectorParamsAs1DForOutWhenUnconnected=off
  wires:
  In1/1 -> MATLAB Function1/2(state)
  Constant/1 -> MATLAB Function1/3(rangeSensorLocBody)
  Constant1/1 -> MATLAB Function1/4(rangeSensorAngBody)
  Constant2/1 -> MATLAB Function1/5(rangeSensorFOV)
  MATLAB Function1/1(range) -> range/1
  Constant3/1 -> MATLAB Function1/6(wallBounds)
  MATLAB Function1/2(rangeArray) -> rangeArray/1
  Time/1 -> MATLAB Function1/1(t)

== system AirTableModel/Executive/Guidance ==
  navState : Inport
  refTraj : Inport  Port=2
  GNCMode : Inport  Port=3
  Time : Inport  Port=4
  controlType : Inport  Port=5
  rangeData : Inport  Port=6
  Multiport Switch1 : MultiPortSwitch  Inputs=2
  RangeSensorGuidance : Subsystem
  ReferenceTrajectoryGuidance : Subsystem
  Selector : Selector  InputPortWidth=12  IndexOptions=Index vector (dialog)  Indices=[4:12]  OutputSizes=1
  Vector Concatenate : Concatenate
  Out1 : Outport
  wires:
  Time/1 -> ReferenceTrajectoryGuidance/1(Time)
  ReferenceTrajectoryGuidance/1(referenceValues) -> Selector/1, Multiport Switch1/2
  refTraj/1 -> ReferenceTrajectoryGuidance/2(refTraj)
  GNCMode/1 -> Multiport Switch1/1
  controlType/1 -> ReferenceTrajectoryGuidance/3(controlType)
  Multiport Switch1/1 -> Out1/1
  Selector/1 -> Vector Concatenate/2
  Vector Concatenate/1 -> Multiport Switch1/3
  navState/1 -> RangeSensorGuidance/1(In1)
  rangeData/1 -> RangeSensorGuidance/2(rangeSensorData)
  RangeSensorGuidance/1(desiredPosECEF) -> Vector Concatenate/1

== system AirTableModel/Navigation/ComputeVelocity ==
  Position : Inport
  Discrete Derivative : simulink/Discrete/Discrete Derivative  gainval=1.0  ICPrevScaledInput=0.0  OutMin=[]  OutMax=[]  OutDataType=fixdt(1, 16)  OutScaling=2^-10  DoSatur=off
  ProcessedVelocity : Outport  VectorParamsAs1DForOutWhenUnconnected=off
  wires:
  Position/1 -> Discrete Derivative/1
  Discrete Derivative/1 -> ProcessedVelocity/1

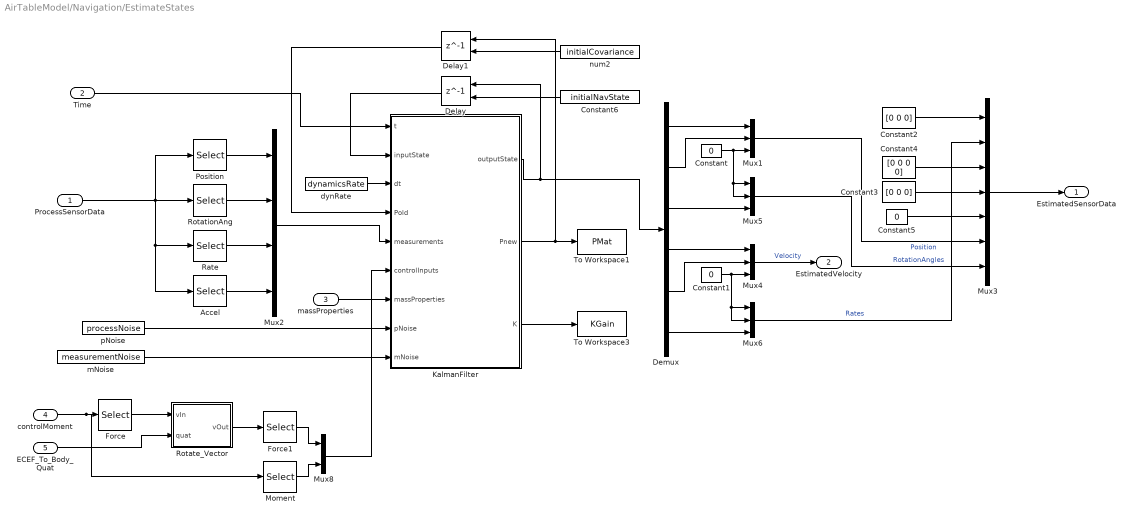
== system AirTableModel/Navigation/EstimateStates ==
  ProcessSensorData : Inport
  Time : Inport  Port=2
  massProperties : Inport  Port=3
  controlMoment : Inport  Port=4
  ECEF_To_Body_Quat : Inport  Port=5
  Accel : Selector  InputPortWidth=20  IndexOptions=Index vector (dialog)  Indices=[1:2]  OutputSizes=1
  Constant : Constant  Value=0
  Constant1 : Constant  Value=0
  Constant2 : Constant  Value=[0 0 0]
  Constant3 : Constant  Value=[0 0 0]
  Constant4 : Constant  Value=[0 0 0 0]
  Constant5 : Constant  Value=0
  Constant6 : Constant  Value=initialNavState
  Delay : Delay  DelayLength=1  InitialConditionSource=Input port
      settings: InputPortMap=u0,p4
  Delay1 : Delay  DelayLength=1  InitialConditionSource=Input port
      settings: InputPortMap=u0,p4
  Demux : Demux  Outputs=6
  Force : Selector  InputPortWidth=6  IndexOptions=Index vector (dialog)  Indices=[1:3]  OutputSizes=1
  Force1 : Selector  InputPortWidth=3  IndexOptions=Index vector (dialog)  Indices=[1:2]  OutputSizes=1
  KalmanFilter : MATLAB Function  TreatAsAtomicUnit=on
  Moment : Selector  InputPortWidth=6  IndexOptions=Index vector (dialog)  Indices=6  OutputSizes=1
  Mux{1,4..6} (4 alike) : Mux  Inputs=3
  Mux2 : Mux
  Mux3 : Mux  Inputs=7
  Mux8 : Mux  Inputs=2
  Position : Selector  InputPortWidth=20  IndexOptions=Index vector (dialog)  Indices=[15:16]  OutputSizes=1
  Rate : Selector  InputPortWidth=20  IndexOptions=Index vector (dialog)  Indices=[6]  OutputSizes=1
  Rotate_Vector : MATLAB Function  TreatAsAtomicUnit=on
  RotationAng : Selector  InputPortWidth=20  IndexOptions=Index vector (dialog)  Indices=[20]  OutputSizes=1
  To Workspace1 : ToWorkspace  VariableName=PMat  SaveFormat=Timeseries  SampleTime=-1
  To Workspace3 : ToWorkspace  VariableName=KGain  SaveFormat=Timeseries  SampleTime=-1
  dynRate : Constant  Value=dynamicsRate  VectorParams1D=off
  mNoise : Constant  Value=measurementNoise  VectorParams1D=off
  num2 : Constant  Value=initialCovariance  VectorParams1D=off
  pNoise : Constant  Value=processNoise  VectorParams1D=off
  EstimatedSensorData : Outport  VectorParamsAs1DForOutWhenUnconnected=off
  EstimatedVelocity : Outport  Port=2  VectorParamsAs1DForOutWhenUnconnected=off
  wires:
  Mux3/1 -> EstimatedSensorData/1
  ProcessSensorData/1 -> Position/1, Rate/1, Accel/1, RotationAng/1
  KalmanFilter/1(outputState) -> Demux/1, Delay/1
  Delay/1 -> KalmanFilter/2(inputState)
  KalmanFilter/2(Pnew) -> To Workspace1/1, Delay1/1
  Delay1/1 -> KalmanFilter/4(Pold)
  Position/1 -> Mux2/1
  RotationAng/1 -> Mux2/2
  Rate/1 -> Mux2/3
  Accel/1 -> Mux2/4
  Mux2/1 -> KalmanFilter/5(measurements)
  num2/1 -> Delay1/2
  pNoise/1 -> KalmanFilter/8(pNoise)
  mNoise/1 -> KalmanFilter/9(mNoise)
  massProperties/1 -> KalmanFilter/7(massProperties)
  Demux/1 -> Mux1/1
  Demux/2 -> Mux1/2
  Constant/1 -> Mux5/2, Mux5/1, Mux1/3
  Mux1/1 -> Mux3/6  "Position"
  Demux/4 -> Mux4/1
  Demux/5 -> Mux4/2
  Constant1/1 -> Mux6/2, Mux6/1, Mux4/3
  Mux4/1 -> EstimatedVelocity/1  "Velocity"
  Constant3/1 -> Mux3/4
  Constant4/1 -> Mux3/3
  Constant5/1 -> Mux3/5
  Demux/3 -> Mux5/3
  Mux5/1 -> Mux3/7  "RotationAngles"
  Demux/6 -> Mux6/3
  Mux6/1 -> Mux3/2  "Rates"
  Constant6/1 -> Delay/2
  controlMoment/1 -> Moment/1, Force/1
  Force/1 -> Rotate_Vector/1(vIn)
  ECEF_To_Body_Quat/1 -> Rotate_Vector/2(quat)
  Rotate_Vector/1(vOut) -> Force1/1
  Moment/1 -> Mux8/2
  Force1/1 -> Mux8/1
  Mux8/1 -> KalmanFilter/6(controlInputs)
  Time/1 -> KalmanFilter/1(t)
  KalmanFilter/3(K) -> To Workspace3/1
  dynRate/1 -> KalmanFilter/3(dt)
  Constant2/1 -> Mux3/1

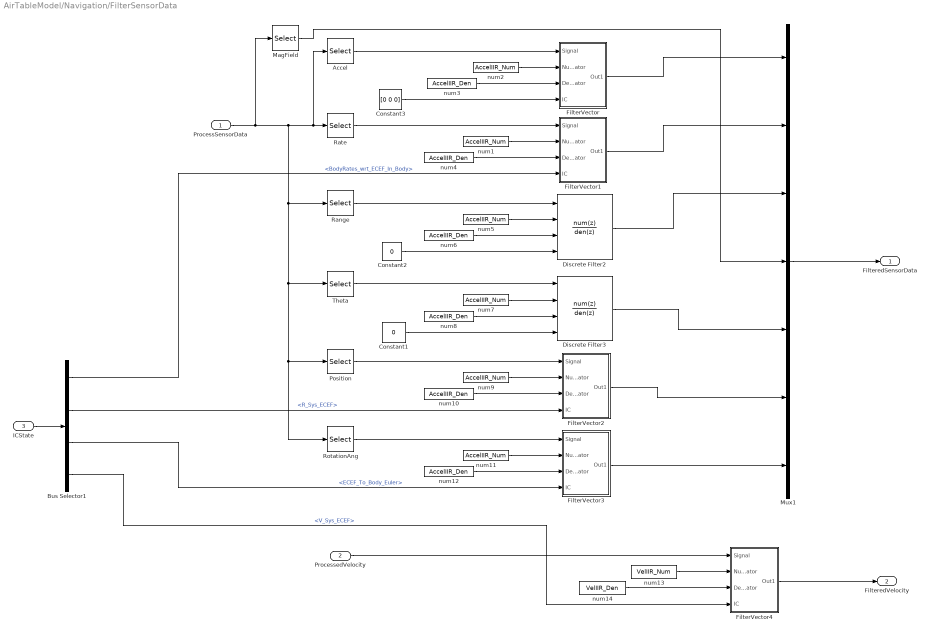
== system AirTableModel/Navigation/FilterSensorData ==
  ProcessSensorData : Inport
  ProcessedVelocity : Inport  Port=2
  ICState : Inport  Port=3
  Accel : Selector  InputPortWidth=20  IndexOptions=Index vector (dialog)  Indices=[1:3]  OutputSizes=1
  Bus Selector1 : BusSelector  OutputSignals=RotState_Body_ECEF.BodyRates_wrt_ECEF_In_Body,TranState_ECEF.R_Sys_ECEF,RotState_Body_ECEF.ECEF_To_Body_Euler,TranState_ECEF.V_Sys_ECEF
  Constant1 : Constant  Value=0
  Constant2 : Constant  Value=0
  Constant3 : Constant  Value=[0 0 0]
  Discrete Filter2 : DiscreteFilter  NumeratorSource=Input port  DenominatorSource=Input port  InitialStatesSource=Input port  a0EqualsOne=on
      settings: InputPortMap=u0,p1,p3,p5
  Discrete Filter3 : DiscreteFilter  NumeratorSource=Input port  DenominatorSource=Input port  InitialStatesSource=Input port  a0EqualsOne=on
      settings: InputPortMap=u0,p1,p3,p5
  FilterVector : Subsystem  TreatAsAtomicUnit=on
      settings: RTWFcnNameOpts=Use subsystem name  RTWFileNameOpts=Use function name
  FilterVector1 : Subsystem  TreatAsAtomicUnit=on
      settings: RTWFcnNameOpts=Use subsystem name  RTWFileNameOpts=Use function name
  FilterVector2 : Subsystem  TreatAsAtomicUnit=on
      settings: RTWFcnNameOpts=Use subsystem name  RTWFileNameOpts=Use function name
  FilterVector3 : Subsystem  TreatAsAtomicUnit=on
      settings: RTWFcnNameOpts=Use subsystem name  RTWFileNameOpts=Use function name
  FilterVector4 : Subsystem  TreatAsAtomicUnit=on
      settings: RTWFcnNameOpts=Use subsystem name  RTWFileNameOpts=Use function name
  MagField : Selector  InputPortWidth=20  IndexOptions=Index vector (dialog)  Indices=[11:13]  OutputSizes=1
  Mux1 : Mux  Inputs=7
  Position : Selector  InputPortWidth=20  IndexOptions=Index vector (dialog)  Indices=[15:17]  OutputSizes=1
  Range : Selector  InputPortWidth=20  IndexOptions=Index vector (dialog)  Indices=[7:10]  OutputSizes=1
  Rate : Selector  InputPortWidth=20  IndexOptions=Index vector (dialog)  Indices=[4:6]  OutputSizes=1
  RotationAng : Selector  InputPortWidth=20  IndexOptions=Index vector (dialog)  Indices=[18:20]  OutputSizes=1
  Theta : Selector  InputPortWidth=20  IndexOptions=Index vector (dialog)  Indices=[14]  OutputSizes=1
  num{1..2,5,7,9,11} (6 alike) : Constant  Value=AccelIIR_Num  VectorParams1D=off
  num{3..4,6,8,10,12} (6 alike) : Constant  Value=AccelIIR_Den  VectorParams1D=off
  num13 : Constant  Value=VelIIR_Num  VectorParams1D=off
  num14 : Constant  Value=VelIIR_Den  VectorParams1D=off
  FilteredSensorData : Outport  VectorParamsAs1DForOutWhenUnconnected=off
  FilteredVelocity : Outport  Port=2  VectorParamsAs1DForOutWhenUnconnected=off
  wires:
  Mux1/1 -> FilteredSensorData/1
  num3/1 -> FilterVector/3(Denominator)
  num2/1 -> FilterVector/2(Numerator)
  FilterVector/1(Out1) -> Mux1/1
  FilterVector1/1(Out1) -> Mux1/2
  MagField/1 -> Mux1/4
  num4/1 -> FilterVector1/3(Denominator)
  num1/1 -> FilterVector1/2(Numerator)
  num6/1 -> Discrete Filter2/3
  num5/1 -> Discrete Filter2/2
  num8/1 -> Discrete Filter3/3
  num7/1 -> Discrete Filter3/2
  num10/1 -> FilterVector2/3(Denominator)
  num9/1 -> FilterVector2/2(Numerator)
  num12/1 -> FilterVector3/3(Denominator)
  num11/1 -> FilterVector3/2(Numerator)
  Discrete Filter2/1 -> Mux1/3
  Discrete Filter3/1 -> Mux1/5
  FilterVector2/1(Out1) -> Mux1/6
  FilterVector3/1(Out1) -> Mux1/7
  Rate/1 -> FilterVector1/1(Signal)
  Range/1 -> Discrete Filter2/1
  Theta/1 -> Discrete Filter3/1
  Position/1 -> FilterVector2/1(Signal)
  num14/1 -> FilterVector4/3(Denominator)
  num13/1 -> FilterVector4/2(Numerator)
  ProcessedVelocity/1 -> FilterVector4/1(Signal)
  FilterVector4/1(Out1) -> FilteredVelocity/1
  RotationAng/1 -> FilterVector3/1(Signal)
  Accel/1 -> FilterVector/1(Signal)
  ProcessSensorData/1 -> RotationAng/1, Position/1, Theta/1, Range/1, Accel/1, Rate/1, MagField/1
  Constant3/1 -> FilterVector/4(IC)
  Constant2/1 -> Discrete Filter2/4
  ICState/1 -> Bus Selector1/1
  Bus Selector1/1 -> FilterVector1/4(IC)  "<BodyRates_wrt_ECEF_In_Body>"
  Bus Selector1/2 -> FilterVector2/4(IC)  "<R_Sys_ECEF>"
  Bus Selector1/3 -> FilterVector3/4(IC)  "<ECEF_To_Body_Euler>"
  Bus Selector1/4 -> FilterVector4/4(IC)  "<V_Sys_ECEF>"
  Constant1/1 -> Discrete Filter3/4

== system AirTableModel/Navigation/FormNewState ==
  navType : Inport
  trueState : Inport  Port=2
  measuredState : Inport  Port=3
  filteredState : Inport  Port=4
  estimatedState : Inport  Port=5
  Multiport Switch : MultiPortSwitch  Inputs=4
  Out3 : Outport  VectorParamsAs1DForOutWhenUnconnected=off
  wires:
  trueState/1 -> Multiport Switch/2
  measuredState/1 -> Multiport Switch/3
  estimatedState/1 -> Multiport Switch/5
  Multiport Switch/1 -> Out3/1
  filteredState/1 -> Multiport Switch/4
  navType/1 -> Multiport Switch/1

== system AirTableModel/Process Inputs/Create Reference Trajectory ==
  PositionData : Inport
  RotationData : Inport  Port=2
  refIdx : Inport  Port=3
  controlType : Inport  Port=4
  ICState : Inport  Port=5
  Enable : EnablePort
  Add : Sum
  Constant : Constant  Value=R_Tracker_To_ECEF
  Constant1 : Constant  Value=M_Tracker_To_Body
  ConvertToMeters : Gain  Gain=1/1000
  ConvertToRadians : Gain  Gain=pi/180
  MATLAB Function1 : MATLAB Function  TreatAsAtomicUnit=on
  Product1 : Product  Multiplication=Matrix(*)
  refTraj : Outport  VectorParamsAs1DForOutWhenUnconnected=off
  wires:
  MATLAB Function1/1(refTraj) -> refTraj/1
  refIdx/1 -> MATLAB Function1/1(refIdx)
  ICState/1 -> MATLAB Function1/2(ICState)
  ConvertToMeters/1 -> Add/2
  PositionData/1 -> MATLAB Function1/5(rawPosition), ConvertToMeters/1
  Constant/1 -> Add/1
  ConvertToRadians/1 -> Product1/2
  Constant1/1 -> Product1/1
  RotationData/1 -> ConvertToRadians/1
  Add/1 -> MATLAB Function1/4(PositionData)
  Product1/1 -> MATLAB Function1/6(RotationData)
  controlType/1 -> MATLAB Function1/3(controlType)

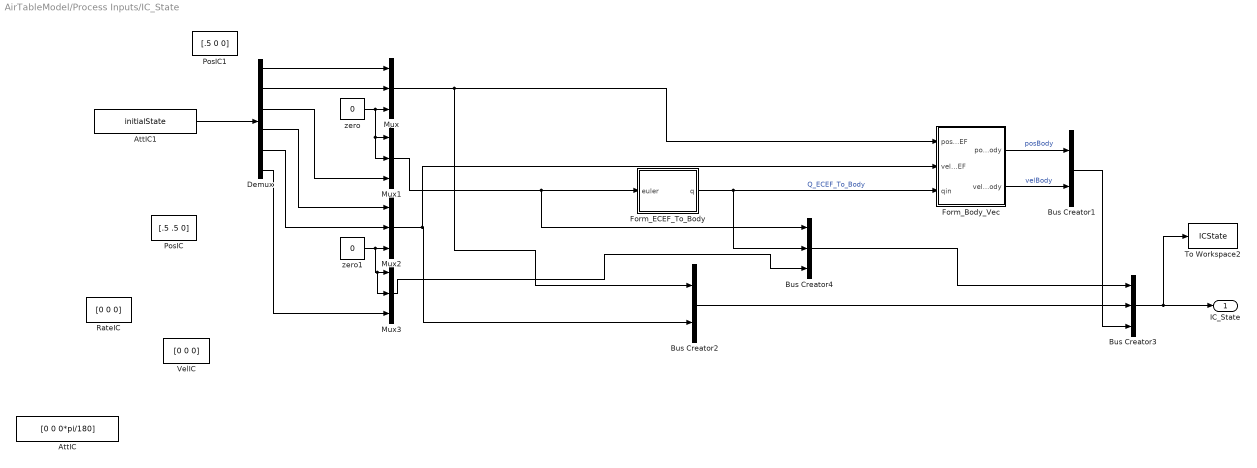
== system AirTableModel/Process Inputs/IC_State ==
  AttIC : Constant  Value=[0 0 0*pi/180]
  AttIC1 : Constant  Value=initialState
  Bus Creator1 : BusCreator  Inputs=2  OutDataTypeStr=Bus: TranStateBodyBus
      settings: InheritFromInputs=off
  Bus Creator2 : BusCreator  Inputs=2  OutDataTypeStr=Bus: TranStateECEFBus
      settings: InheritFromInputs=off
  Bus Creator3 : BusCreator  Inputs=3  OutDataTypeStr=Bus: FullStateBus
      settings: InheritFromInputs=off
  Bus Creator4 : BusCreator  Inputs=3  OutDataTypeStr=Bus: RotStateBodyECEFBus
      settings: InheritFromInputs=off
  Demux : Demux  Outputs=6
  Form_Body_Vec : MATLAB Function  TreatAsAtomicUnit=on
  Form_ECEF_To_Body : MATLAB Function  TreatAsAtomicUnit=on
  Mux{,1..3} (4 alike) : Mux  Inputs=3
  PosIC : Constant  Value=[.5 .5 0]
  PosIC1 : Constant  Value=[.5 0 0]
  RateIC : Constant  Value=[0 0 0]
  To Workspace2 : ToWorkspace  VariableName=ICState  SaveFormat=Timeseries  SampleTime=-1
  VelIC : Constant  Value=[0 0 0]
  zero : Constant  Value=0
  zero1 : Constant  Value=0
  IC_State : Outport  VectorParamsAs1DForOutWhenUnconnected=off
  wires:
  Form_ECEF_To_Body/1(q) -> Form_Body_Vec/3(qin), Bus Creator4/2  "Q_ECEF_To_Body"
  Form_Body_Vec/1(posBody) -> Bus Creator1/1  "posBody"
  Form_Body_Vec/2(velBody) -> Bus Creator1/2  "velBody"
  Bus Creator2/1 -> Bus Creator3/2
  Bus Creator1/1 -> Bus Creator3/3
  Bus Creator4/1 -> Bus Creator3/1
  Bus Creator3/1 -> To Workspace2/1, IC_State/1
  AttIC1/1 -> Demux/1
  Demux/1 -> Mux/1
  Demux/2 -> Mux/2
  zero/1 -> Mux1/2, Mux1/1, Mux/3
  Mux/1 -> Bus Creator2/1, Form_Body_Vec/1(posECEF)
  Demux/3 -> Mux1/3
  Mux1/1 -> Form_ECEF_To_Body/1(euler), Bus Creator4/1
  Demux/4 -> Mux2/1
  Demux/5 -> Mux2/2
  zero1/1 -> Mux3/2, Mux3/1, Mux2/3
  Mux2/1 -> Form_Body_Vec/2(velECEF), Bus Creator2/2
  Demux/6 -> Mux3/3
  Mux3/1 -> Bus Creator4/3

== system AirTableModel/Process Inputs/Variant Subsystem ==
  note: 1) Add Subsystem or Model blocks as valid variant choices.
      | 2) You cannot connect blocks at this level. At simulation, connectivity is automatically
      | determined, based on the active variant and port name matching.
  refIdx : Inport
  navType : Inport  Port=2
  controlType : Inport  Port=3  OutDataTypeStr=uint8  PortDimensions=1
  UseInputPorts : Subsystem  VariantControl=VSS_INPUTPORT
  UseWorkspaceData : Subsystem  VariantControl=VSS_WORKSPACEDATA
  refIdxOut : Outport
  navTypeOut : Outport  Port=2
  controlTypeOut : Outport  Port=3

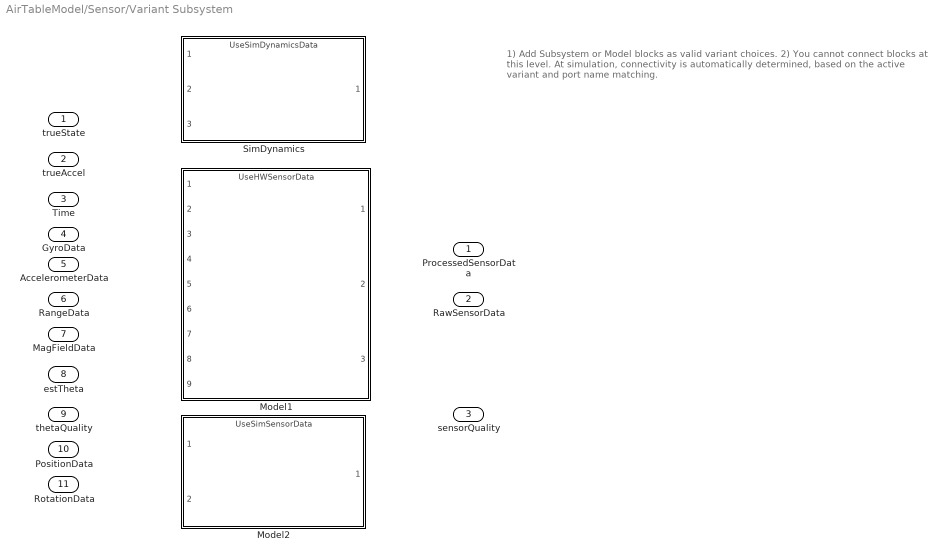
== system AirTableModel/Sensor/Variant Subsystem ==
  note: 1) Add Subsystem or Model blocks as valid variant choices.
      | 2) You cannot connect blocks at this level. At simulation, connectivity is automatically
      | determined, based on the active variant and port name matching.
  trueState : Inport
  trueAccel : Inport  Port=2
  Time : Inport  Port=3  OutDataTypeStr=double
  GyroData : Inport  Port=4
  AccelerometerData : Inport  Port=5
  RangeData : Inport  Port=6  OutDataTypeStr=int32
  MagFieldData : Inport  Port=7
  estTheta : Inport  Port=8
  thetaQuality : Inport  Port=9
  PositionData : Inport  Port=10
  RotationData : Inport  Port=11
  Model1 : ModelReference  ModelNameDialog=UseHWSensorData  SimulationMode=Normal  VariantControl=VSS_HWSENSOR  ModelReferenceVersion=1.152
  Model2 : ModelReference  ModelNameDialog=UseSimSensorData  SimulationMode=Normal  VariantControl=VSS_SIMSENSOR  ModelReferenceVersion=1.28
  SimDynamics : ModelReference  ModelNameDialog=UseSimDynamicsData  SimulationMode=Normal  VariantControl=VSS_SIMDYNAMICS  ModelReferenceVersion=1.43
  ProcessedSensorData : Outport  VectorParamsAs1DForOutWhenUnconnected=off
  RawSensorData : Outport  Port=2  VectorParamsAs1DForOutWhenUnconnected=off
  sensorQuality : Outport  Port=3  VectorParamsAs1DForOutWhenUnconnected=off
